simulink model "week3_problem1"  (R2019b)
settings: Solver=VariableStepAuto  StartTime=0.0  StopTime=10.0  RelTol=1e-3
settings Model: Creator=Shreyas  LastModifiedBy=Shreyas

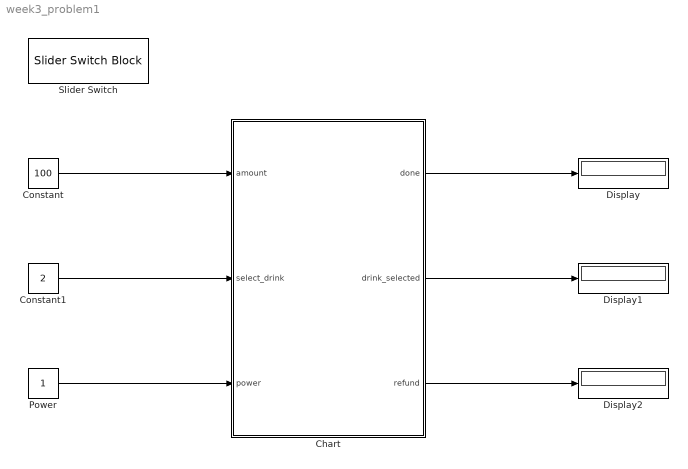
== system week3_problem1 ==
  Chart : Stateflow chart  TreatAsAtomicUnit=on
  Constant : Constant  Value=100
  Constant1 : Constant  Value=2
  Display : Display
  Display1 : Display
  Display2 : Display
  Power : Constant
  Slider Switch : SliderSwitchBlock
      settings: Values={{'Off', 'On'}, [0 1]}
  wires:
  Power/1 -> Chart/3(power)
  Chart/3(refund) -> Display2/1
  Chart/1(done) -> Display/1
  Constant/1 -> Chart/1(amount)
  Chart/2(drink_selected) -> Display1/1
  Constant1/1 -> Chart/2(select_drink)

== stateflow chart week3_problem1/Chart ==
  data: drink_cost local =10; done output =0; amount input; select_drink input; drink_selected output; refund output; power input
